simulink library "inp"  (Simulink 7.4)
settings: Solver=ode45  StartTime=0.0  StopTime=10.0  RelTol=1e-3
undefined symbols (not defined in the file): AINP_BrkPedalInterp_X_bar, C_TASK_10MS_S, ENUM_SHIFTER_D, ENUM_SHIFTER_N, ENUM_SHIFTER_P, ENUM_SHIFTER_R, KINP_BonnetCloseVehSpdThre_kph, KINP_EDUCoolantTempFilTm_s, KINP_EDUOilPressureFilTm_s, KINP_EDUOilTempFilTm_s, KINP_EDUSynchDisp_mm, KINP_EDUSynchPosnPWMDC_pct_LowerLimit, KINP_EDUSynchPosnPWMDC_pct_ovrdflg, KINP_EDUSynchPosnPWMDC_pct_ovrdval, KINP_EDUSynchPosnPWMDC_pct_UpperLimit, KINP_ShifterPosConfirmD_s, KINP_ShifterPosConfirmN_s, KINP_ShifterPosConfirmP_s, KINP_ShifterPosConfirmR_s, KINP_SingleAccPedalFltRateLim_pct, KINP_TMSpd2VehSpdSigNeg_rpm, KINP_TMSpd2VehSpdSigPos_rpm, KINP_ValidCheck_EDUSynchPosnPWMDC_dec, KINP_ValidCheck_EDUSynchPosnPWMDC_inc, KINP_ValidCheck_EDUSynchPosnPWMDC_lim, KINP_VehSpdSigKeepThres_kph, KPH2MPS, MIN2SEC, MINP_BrkPedalInterp_pct, MPS2KPH, PI, seat_version_control_block_callbacks, TIRE_RADIUS
libraries: inp_lib x166, hcu_lib x4, simulink x1
(part 1 of 9)
settings Model: Creator=tunfl  LastModifiedBy=tunfl
settings Model: ModifiedHistory=|
  | Function: INP
  | Version: 11.0.9
  | Time: 2012-08-28 16:30:24
  | By: tunfl
  | 0036:ACR_INP_0006:INP: Filter process change about shifter position
  | 
  | 
  | Function: INP
  | Version: 11.0.10
  | Time: 2012-09-03 11:55:18
  | By: tunfl
  | Bug fix for Mantis2038(ACR_INP_0006): Deleted VSRV_ShifterPosValid_ovrdflg&VSRV_ShifterPosValid_ovrdval
  | 
  | 
  | Function: INP
  | Version: 11.0.11
  | Time: 2012-10-10 16:30:31
  | By: tunfl
  | Mantis 2033: Added increasing filter for accelerate pedal position
  | 
  | 
  | Function: INP
  | Version: 11.0.12
  | Time: 2012-10-11 11:20:51
  | By: tunfl
  | Mantis 2079: Newly add signals:VINP_TMOverTemp_flg && VINP_ISGOverTemp_flg
  | 
  | 
  | Function: INP
  | Version: 11.0.13
  | Time: 2012-10-11 11:22:44
  | By: tunfl
  | Mantis 2078: Newly add new signals: VINP_TMDerating_flg && VINP_ISGDerating_flg
  | 
  | 
  | Function: INP
  | Version: 11.0.14
  | Time: 2012-10-16 14:48:04
  | By: tunfl
  | Fixed Library-Link problem for signal: VINP_ShifterPosValid_flg
  | 
  | 
  | Function: INP
  | Version: 11.0.15
  | Time: 2012-10-19 16:16:11
  | By: tunfl
  | Added a new signal: VHAL_ShifterPosProtFault_flg
  | 
  | 
  | Function: INP
  | Version: 11.0.16
  | Time: 2012-11-23 11:36:28
  | By: tunfl
  | Fixed the missing GoTo label problem.
  | 
  | 
  | Function: INP
  | Version: 11.0.17
  | Time: 2012-12-04 09:11:36
  | By: tunfl
  | Changed MAX/MIN value of ISGSpeed to +/-7000
  | 
  | 
  | Function: INP
  | Version: 11.0.18
  | Time: 2013-03-15 10:45:21
  | By: wuqnj
  | Mantis 002142(RSC_INP_0007) and 002147(RSC_INP_0008): New simplification library and CAN MsgActive signals are derived from DSM rather than HAL lay.
  | 
  | 
  | Function: INP
  | Version: 11.0.22
  | Time: 2013-03-19 10:45:50
  | By: wuqnj
  | Add signals into INP fit for v1.7 dbc definition.
  | 
  | 
  | Function: INP
  | Version: 11.0.25
  | Time: 2013-04-10 13:18:30
  | By: wuqnj
  | Add the signals display in INCA for VINP_ISGPwrAct_kW and VINP_ISGOffsetAng_deg
  | 
  | 
  | Function: INP
  | Version: 11.0.26
  | Time: 2013-04-22 16:40:45
  | By: tunfl
  | Changed the improper name of some variables, e.g.  message active signals are started with 'VHAL'
  | 
  | 
  | Function: INP
  | Version: 11.0.28
  | Time: 2013-07-25 13:52:57
  | By: tunfl
  | Mantis_2320: INP/PMM: SCU protection fault should be taken into consideration when determining SCU message is active or not
  | 
  | 
  | Function: INP
  | Version: 11.0.29
  | Time: 2013-08-02 09:13:15
  | By: tunfl
  | Break link with timer library.
  | 
  | 
  | Function: INP
  | Version: 11.0.30
  | Time: 2013-08-05 11:11:04
  | By: tunfl
  | Mantis_2323:INP: Several hardwired signals is processed with first order filter.(EDU Oil pressure, coolant temp, oil temp)

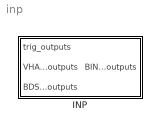
== system inp ==
  INP : Subsystem

== system inp/INP ==
  trig_outputs : Inport
  VHAL_outputs : Inport  Port=2  UseBusObject=on
      settings: BusObject=BHAL_outputs
  BDSM_outputs : Inport  Port=3
  Bus Creator : BusCreator  Inputs=3
  Bus Creator2 : BusCreator  Inputs=5
  Bus Selector : BusSelector  OutputSignals=trig_inp_5ms,trig_inp_10ms,trig_inp_20ms,trig_inp_50ms,trig_inp_100ms
  Bus Selector2 : BusSelector  OutputSignals=VHAL_outputs_5ms,VHAL_outputs_10ms,VHAL_outputs_20ms,VHAL_outputs_50ms,VHAL_outputs_100ms
  Chart : Stateflow chart  RTWFcnName=INP_5MS  RTWFileName=INP
      settings: RTWSystemCode=Function  RTWFcnNameOpts=User specified  RTWFileNameOpts=User specified
  Chart1 : Stateflow chart  RTWFcnName=INP_5MS  RTWFileName=INP
      settings: RTWSystemCode=Inline  RTWFcnNameOpts=User specified  RTWFileNameOpts=User specified
  INP_100MS : Subsystem  TreatAsAtomicUnit=on  RTWFcnName=INP_100MS  RTWFileName=INP
      settings: RTWSystemCode=Function  RTWFcnNameOpts=User specified  RTWFileNameOpts=User specified
  INP_10MS : Subsystem  TreatAsAtomicUnit=on  RTWFcnName=INP_10MS  RTWFileName=INP
      settings: RTWSystemCode=Function  RTWFcnNameOpts=User specified  RTWFileNameOpts=User specified
  INP_20MS : Subsystem  TreatAsAtomicUnit=on  RTWFcnName=INP_20MS  RTWFileName=INP
      settings: RTWSystemCode=Function  RTWFcnNameOpts=User specified  RTWFileNameOpts=User specified
  INP_50MS : Subsystem  TreatAsAtomicUnit=on  RTWFcnName=INP_50MS  RTWFileName=INP
      settings: RTWSystemCode=Function  RTWFcnNameOpts=User specified  RTWFileNameOpts=User specified
  INP_5MS : Subsystem  TreatAsAtomicUnit=on
  INP_MsgAlive_flg : Subsystem  TreatAsAtomicUnit=on  RTWFcnName=INP_MsgAlive_flg  RTWFileName=INP
      settings: RTWSystemCode=Inline  RTWFcnNameOpts=User specified  RTWFileNameOpts=User specified
  Pre-Process : Subsystem
  Version_Control : Subsystem  LoadFcn=seat_version_control_block_callbacks(gcb,'load');  mask(SEAT_Version_Control){version=11.0.30, b_submit_to_excel=on, function_type=Sub, function_name=INP, record_file_name=INP_VersionControl.xlsx, version_on_load=11.0.30, version_last_saved=11.0.30, file_bytes_on_load=1788854, file_date_on_load=735451.46667824069, file_name_on_load=inp.mdl}
      mask prompts: b_submit_to_excel "Submit to record file"; function_type "Function Type"; function_name "Function Name"; record_file_name "Record File"; file_name_on_load "Mask Parameter 11:"
      mask help:
      | Used to record model and software versions for EP11
      | 1. Version display
      | 2. Submit model change to the target record file (file location could be customized in the "Setting" tab)
      settings: ModelCloseFcn=seat_version_control_block_callbacks(gcb,'modelclose')
      mask StyleString: edit,checkbox,popup(Main|Sub),edit,edit,edit,edit,edit,edit,edit
      mask TabNameString: Version,Version,Setting,Setting,Setting,Setting,Setting,Setting,Setting,Setting
      mask Display: disp(sprintf('Function: \t%s\nVersion: \t%s',function_name,version))
  BINP_outputs : Outport  UseBusObject=on
      settings: BusObject=BINP_outputs
  wires:
  [BDSM_outputs] -> Pre-Process/3(BDSM_outputs)
  [trig_can_msg_alive_10ms] -> INP_MsgAlive_flg/Trigger  "fcn_call"
  Chart1/2(trig_can_msg_alive_10ms) -> [trig_can_msg_alive_10ms]
  Chart1/1(trig_inp_raw_10ms) -> [trig_inp_raw_10ms]
  [trig_inp_10ms] -> Chart1/Trigger
  [BINP_CANMsgAlive] -> INP_20MS/2(BINP_CANMsgAlive)
  [BINP_CANMsgAlive] -> INP_50MS/2(BINP_CANMsgAlive)
  [BINP_CANMsgAlive] -> INP_100MS/2(BINP_CANMsgAlive)
  [BINP_CANMsgAlive] -> INP_10MS/2(BINP_CANMsgAlive)
  INP_MsgAlive_flg/1(BINP_CANMsgAlive) -> [BINP_CANMsgAlive]
  BDSM_outputs/1 -> [BDSM_outputs], INP_MsgAlive_flg/1(BDSM_outputs)
  Bus Creator/1 -> [trig_sig_chk]
  Chart/4(trig_sig_chk_100ms) -> Bus Creator/3
  Chart/3(trig_sig_chk_10ms) -> Bus Creator/2
  [trig_sig_chk] -> Pre-Process/1(trig_sig_chk)
  Bus Selector/5 -> [trig_inp_100ms]  "<trig_inp_100ms>"
  Bus Selector/4 -> [trig_inp_50ms]  "<trig_inp_50ms>"
  Bus Selector/3 -> [trig_inp_20ms]  "<trig_inp_20ms>"
  Bus Selector/2 -> [trig_inp_10ms]  "<trig_inp_10ms>"
  Bus Selector/1 -> [trig_inp_5ms]  "<trig_inp_5ms>"
  trig_outputs/1 -> Bus Selector/1
  VHAL_outputs/1 -> Bus Selector2/1
  Bus Creator2/1 -> Pre-Process/2(BINP_rawoutputs)  "BINP_rawoutputs"
  Pre-Process/1(BINP_outputs) -> BINP_outputs/1  "BINP_outputs"
  [trig_inp_100ms] -> INP_100MS/Trigger
  [trig_inp_50ms] -> INP_50MS/Trigger
  [trig_inp_20ms] -> INP_20MS/Trigger
  [trig_inp_raw_10ms] -> INP_10MS/Trigger
  Bus Selector2/1 -> INP_5MS/1(BHAL_IN5MS)  "<VHAL_outputs_5ms>"
  INP_5MS/1(BINP_rawoutputs_5ms) -> Bus Creator2/1
  INP_100MS/1(BINP_rawoutputs_100ms) -> Bus Creator2/5
  INP_50MS/1(BINP_rawoutputs_50ms) -> Bus Creator2/4
  INP_20MS/1(BINP_rawoutputs_20ms) -> Bus Creator2/3
  INP_10MS/1(BINP_rawoutputs_10ms) -> Bus Creator2/2
  Bus Selector2/5 -> INP_100MS/1(BHAL_IN_100ms)  "<VHAL_outputs_100ms>"
  Bus Selector2/4 -> INP_50MS/1(BHAL_IN_50ms)  "<VHAL_outputs_50ms>"
  Bus Selector2/3 -> INP_20MS/1(BHAL_IN_20ms)  "<VHAL_outputs_20ms>"
  Bus Selector2/2 -> INP_10MS/1(BHAL_IN_10ms)  "<VHAL_outputs_10ms>"
  Chart/1(trig_5ms_raw) -> [trig_5ms_raw]
  Chart/2(trig_sig_chk_5ms) -> Bus Creator/1
  [trig_5ms_raw] -> INP_5MS/Trigger
  [trig_inp_5ms] -> Chart/Trigger

== system inp/INP/INP_100MS ==
  BHAL_IN_100ms : Inport  OutDataType=fixdt(1, 16)  OutScaling=2^0
  BINP_CANMsgAlive : Inport  Port=2  OutDataType=fixdt(1, 16)  OutScaling=2^0
  INP_100MS_fcn_call : TriggerPort  TriggerType=function-call
  BSRV_In_ovrdflgs : Subsystem
  BSRV_in_ovrdvals : Subsystem
  Bus Creator3 : BusCreator  Inputs=9
  Bus Selector1 : BusSelector  OutputSignals=VINP_ISCMsgAlive_flg
  Bus Selector14 : BusSelector  OutputSignals=VINP_SMUMsgAlive_flg
  Bus Selector3 : BusSelector  OutputSignals=VINP_TCMsgAlive_flg
  Bus Selector4 : BusSelector  OutputSignals=VINP_ISCMsgAlive_flg
  Bus Selector5 : BusSelector  OutputSignals=VINP_ISCMsgAlive_flg
  Bus Selector7 : BusSelector  OutputSignals=VINP_PMUMsgAlive_flg
  Bus Selector8 : BusSelector  OutputSignals=VINP_SMUMsgAlive_flg
  Bus Selector9 : BusSelector  OutputSignals=VINP_SMUMsgAlive_flg
  HW_HCU_100ms : Subsystem
  Message (100ms) ISC_HSC2_FrP01 : Subsystem
  Message (100ms) ISC_HSC2_FrP02 : Subsystem
  Message (100ms) ISC_HSC2_FrP05 : Subsystem
  Message (100ms) PMU_HSC_FrP00 : Subsystem
  Message (100ms) SMU_HSC_FrP06 : Subsystem
  Message (100ms) SMU_HSC_FrP07 : Subsystem
  Message (100ms) TC_HSC2_FrP03 : Subsystem
  Message (90ms) SMU_HSC_FrP00 : Subsystem
  BINP_rawoutputs_100ms : Outport  OutDataType=fixdt(1, 16)  OutScaling=2^0
  wires:
  [MsgAlive] -> Bus Selector14/1
  [MsgAlive] -> Bus Selector9/1
  [MsgAlive] -> Bus Selector8/1
  [MsgAlive] -> Bus Selector7/1
  [MsgAlive] -> Bus Selector5/1
  [MsgAlive] -> Bus Selector4/1
  [MsgAlive] -> Bus Selector3/1
  [MsgAlive] -> Bus Selector1/1
  BINP_CANMsgAlive/1 -> [MsgAlive]
  Bus Selector5/1 -> Message (100ms) ISC_HSC2_FrP02/4(VINP_ISCMsgAlive_flg)  "<VINP_ISCMsgAlive_flg>"
  HW_HCU_100ms/1(BINP_HW_HCU_100ms) -> Bus Creator3/9
  [BSRV_In_ovrdvals] -> HW_HCU_100ms/3(BSRV_In_ovrdvals)
  [BSRV_In_ovrdflgs] -> HW_HCU_100ms/2(BSRV_In_ovrdflgs)
  Message (90ms) SMU_HSC_FrP00/1(BINP_SMU_HSC_FrP00) -> Bus Creator3/8
  Message (100ms) SMU_HSC_FrP07/1(BINP_SMU_HSC_FrP07) -> Bus Creator3/7
  Message (100ms) SMU_HSC_FrP06/1(BINP_SMU_HSC_FrP06) -> Bus Creator3/6
  Message (100ms) PMU_HSC_FrP00/1(BINP_PMU_HSC_FrP00) -> Bus Creator3/5
  BSRV_in_ovrdvals/1(output_bus) -> [BSRV_In_ovrdvals]
  BSRV_In_ovrdflgs/1(output_bus) -> [BSRV_In_ovrdflgs]
  Bus Creator3/1 -> BINP_rawoutputs_100ms/1  "BINP_rawoutputs_100ms"
  [BSRV_In_ovrdvals] -> Message (100ms) SMU_HSC_FrP07/3(BSRV_In_ovrdvals)
  [BSRV_In_ovrdflgs] -> Message (100ms) SMU_HSC_FrP07/2(BSRV_In_ovrdflgs)
  Bus Selector9/1 -> Message (100ms) SMU_HSC_FrP07/4(VINP_SMUMsgAlive_flg)  "<VINP_SMUMsgAlive_flg>"
  [BSRV_In_ovrdvals] -> Message (100ms) SMU_HSC_FrP06/3(BSRV_In_ovrdvals)
  [BSRV_In_ovrdflgs] -> Message (100ms) SMU_HSC_FrP06/2(BSRV_In_ovrdflgs)
  Bus Selector8/1 -> Message (100ms) SMU_HSC_FrP06/4(VINP_SMUMsgAlive_flg)  "<VINP_SMUMsgAlive_flg>"
  Bus Selector7/1 -> Message (100ms) PMU_HSC_FrP00/4(VINP_PMUMsgAlive_flg)  "<VINP_PMUMsgAlive_flg>"
  [BSRV_In_ovrdvals] -> Message (100ms) PMU_HSC_FrP00/3(BSRV_In_ovrdvals)
  [BSRV_In_ovrdflgs] -> Message (100ms) PMU_HSC_FrP00/2(BSRV_In_ovrdflgs)
  [BSRV_In_ovrdvals] -> Message (100ms) ISC_HSC2_FrP02/3(BSRV_In_ovrdvals)
  [BSRV_In_ovrdflgs] -> Message (100ms) ISC_HSC2_FrP02/2(BSRV_In_ovrdflgs)
  [BSRV_In_ovrdvals] -> Message (100ms) ISC_HSC2_FrP01/3(BSRV_In_ovrdvals)
  [BSRV_In_ovrdflgs] -> Message (100ms) ISC_HSC2_FrP01/2(BSRV_In_ovrdflgs)
  Bus Selector4/1 -> Message (100ms) ISC_HSC2_FrP01/4(VINP_ISCMsgAlive_flg)  "<VINP_ISCMsgAlive_flg>"
  [BSRV_In_ovrdvals] -> Message (100ms) TC_HSC2_FrP03/3(BSRV_In_ovrdvals)
  [BSRV_In_ovrdflgs] -> Message (100ms) TC_HSC2_FrP03/2(BSRV_In_ovrdflgs)
  Bus Selector3/1 -> Message (100ms) TC_HSC2_FrP03/4(VINP_TCMsgAlive_flg)  "<VINP_TCMsgAlive_flg>"
  Bus Selector1/1 -> Message (100ms) ISC_HSC2_FrP05/4(VINP_ISCMsgAlive_flg)  "<VINP_ISCMsgAlive_flg>"
  [BSRV_In_ovrdvals] -> Message (100ms) ISC_HSC2_FrP05/3(BSRV_In_ovrdvals)
  [BSRV_In_ovrdflgs] -> Message (100ms) ISC_HSC2_FrP05/2(BSRV_In_ovrdflgs)
  Bus Selector14/1 -> Message (90ms) SMU_HSC_FrP00/4(VINP_SMUMsgAlive_flg)  "<VINP_SMUMsgAlive_flg>"
  [BSRV_In_ovrdflgs] -> Message (90ms) SMU_HSC_FrP00/2(BSRV_In_ovrdflgs)
  [BSRV_In_ovrdvals] -> Message (90ms) SMU_HSC_FrP00/3(BSRV_In_ovrdvals)
  Message (100ms) ISC_HSC2_FrP05/1(BINP_ISC_HSC2_FrP05) -> Bus Creator3/1
  Message (100ms) TC_HSC2_FrP03/1(BINP_TC_HSC2_FrP03) -> Bus Creator3/2
  Message (100ms) ISC_HSC2_FrP01/1(BINP_ISC_HSC2_FrP01) -> Bus Creator3/3
  Message (100ms) ISC_HSC2_FrP02/1(BINP_ISC_HSC2_FrP02) -> Bus Creator3/4
  BHAL_IN_100ms/1 -> HW_HCU_100ms/1(BHAL_IN_100ms), Message (90ms) SMU_HSC_FrP00/1(BHAL_IN_100ms), Message (100ms) SMU_HSC_FrP07/1(BHAL_IN_100ms), Message (100ms) SMU_HSC_FrP06/1(BHAL_IN_100ms), Message (100ms) PMU_HSC_FrP00/1(BHAL_IN_100ms), Message (100ms) ISC_HSC2_FrP02/1(BHAL_IN_100ms), Message (100ms) ISC_HSC2_FrP01/1(BHAL_IN_100ms), Message (100ms) TC_HSC2_FrP03/1(BHAL_IN_100ms), Message (100ms) ISC_HSC2_FrP05/1(BHAL_IN_100ms)

== system inp/INP/INP_10MS ==
  BHAL_IN_10ms : Inport  OutDataType=fixdt(1, 16)  OutScaling=2^0
  BINP_CANMsgAlive : Inport  Port=2  OutDataType=fixdt(1, 16)  OutScaling=2^0
  INP_10MS_fcn_call : TriggerPort  TriggerType=function-call
  BSRV_in_ovrdflgs : Subsystem
  BSRV_in_ovrdvals : Subsystem
  Bus Creator : BusCreator  Inputs=12
  Bus Selector1 : BusSelector  OutputSignals=VINP_ISCMsgAlive_flg
  Bus Selector{5,8..9,11} (4 alike) : BusSelector  OutputSignals=VINP_DSCMsgAlive_flg
  Bus Selector12 : BusSelector  OutputSignals=VINP_TCMsgAlive_flg
  Bus Selector13 : BusSelector  OutputSignals=VINP_ISCMsgAlive_flg
  Bus Selector2 : BusSelector  OutputSignals=VINP_TCMsgAlive_flg
  Bus Selector3 : BusSelector  OutputSignals=VINP_EMSMsgAlive_flg
  Bus Selector4 : BusSelector  OutputSignals=VINP_EMSMsgAlive_flg
  Bus Selector7 : BusSelector  OutputSignals=VINP_SCUMsgAlive_flg
  HW_HCU_10ms : Subsystem
  Message (10ms) ABS_DSC_HSC_FrP00 : Subsystem
  Message (10ms) ABS_DSC_HSC_FrP03 : Subsystem
  Message (10ms) EMS_HSC_FrP00 : Subsystem
  Message (10ms) EMS_HSC_FrP07 : Subsystem
  Message (10ms) ISC_HSC2_FrP03 : Subsystem
  Message (10ms) ISC_HSC2_FrP04 : Subsystem
  Message (10ms) SCU_HSC_FrP00 : Subsystem
  Message (10ms) TC_HSC2_FrP01 : Subsystem
  Message (10ms) TC_HSC2_FrP02 : Subsystem
  Message (10ms)DSC_HSC_FrP00 : Subsystem
  Message (10ms)DSC_HSC_FrP02 : Subsystem
  BINP_rawoutputs_10ms : Outport  OutDataType=fixdt(1, 16)  OutScaling=2^0
  wires:
  [MsgAlive] -> Bus Selector1/1
  [MsgAlive] -> Bus Selector5/1
  [MsgAlive] -> Bus Selector8/1
  [MsgAlive] -> Bus Selector9/1
  [MsgAlive] -> Bus Selector7/1
  [MsgAlive] -> Bus Selector11/1
  [MsgAlive] -> Bus Selector12/1
  [MsgAlive] -> Bus Selector13/1
  [MsgAlive] -> Bus Selector4/1
  [MsgAlive] -> Bus Selector3/1
  [MsgAlive] -> Bus Selector2/1
  BINP_CANMsgAlive/1 -> [MsgAlive]
  HW_HCU_10ms/1(BINP_HW_HCU_10ms) -> Bus Creator/12
  [BSRV_In_ovrdvals] -> HW_HCU_10ms/3(BSRV_In_ovrdvals)
  [BSRV_In_ovrdflgs] -> HW_HCU_10ms/2(BSRV_In_ovrdflgs)
  Bus Selector3/1 -> Message (10ms) EMS_HSC_FrP00/4(VINP_EMSMsgAlive_flg)  "<VINP_EMSMsgAlive_flg>"
  [BSRV_In_ovrdvals] -> Message (10ms) EMS_HSC_FrP00/3(BSRV_In_ovrdvals)
  [BSRV_In_ovrdflgs] -> Message (10ms) EMS_HSC_FrP00/2(BSRV_In_ovrdflgs)
  Message (10ms) ISC_HSC2_FrP04/1(BINP_ISC_HSC2_FrP04) -> Bus Creator/11
  Message (10ms) ISC_HSC2_FrP03/1(BINP_ISC_HSC2_FrP03) -> Bus Creator/10
  Message (10ms) TC_HSC2_FrP01/1(BINP_TC_HSC2_FrP01) -> Bus Creator/9
  Message (10ms) ABS_DSC_HSC_FrP03/1(BINP_ABS_DSC_HSC_FrP03) -> Bus Creator/8
  Message (10ms) SCU_HSC_FrP00/1(BINP_SCU_HSC_FrP00) -> Bus Creator/7
  Message (10ms)DSC_HSC_FrP02/1(BINP_DSC_HSC_FrP02) -> Bus Creator/6
  Message (10ms)DSC_HSC_FrP00/1(BINP_DSC_HSC_FrP00) -> Bus Creator/5
  Message (10ms) ABS_DSC_HSC_FrP00/1(BINP_ABS_DSC_HSC_FrP00) -> Bus Creator/4
  Message (10ms) EMS_HSC_FrP07/1(BINP_EMS_HSC_FrP07) -> Bus Creator/3  "BINP_EMS_HSC_FrP07"
  Message (10ms) EMS_HSC_FrP00/1(BINP_EMS_HSC_FrP00) -> Bus Creator/2
  Message (10ms) TC_HSC2_FrP02/1(BINP_TC_HSC2_FrP02) -> Bus Creator/1
  Bus Selector5/1 -> Message (10ms) ABS_DSC_HSC_FrP00/4(VINP_DSCMsgAlive_flg)  "<VINP_DSCMsgAlive_flg>"
  [BSRV_In_ovrdflgs] -> Message (10ms) ABS_DSC_HSC_FrP00/2(BSRV_In_ovrdflgs)
  [BSRV_In_ovrdvals] -> Message (10ms) ABS_DSC_HSC_FrP00/3(BSRV_In_ovrdvals)
  Bus Selector8/1 -> Message (10ms)DSC_HSC_FrP00/4(VINP_DSCMsgAlive_flg)  "<VINP_DSCMsgAlive_flg>"
  [BSRV_In_ovrdflgs] -> Message (10ms)DSC_HSC_FrP00/2(BSRV_In_ovrdflgs)
  [BSRV_In_ovrdvals] -> Message (10ms)DSC_HSC_FrP00/3(BSRV_In_ovrdvals)
  BSRV_in_ovrdvals/1(output_bus) -> [BSRV_In_ovrdvals]
  BSRV_in_ovrdflgs/1(output_bus) -> [BSRV_In_ovrdflgs]
  Bus Selector13/1 -> Message (10ms) ISC_HSC2_FrP03/4(VINP_ISCMsgAlive_flg)  "<VINP_ISCMsgAlive_flg>"
  [BSRV_In_ovrdflgs] -> Message (10ms) ISC_HSC2_FrP03/2(BSRV_In_ovrdflgs)
  [BSRV_In_ovrdvals] -> Message (10ms) ISC_HSC2_FrP03/3(BSRV_In_ovrdvals)
  Bus Selector12/1 -> Message (10ms) TC_HSC2_FrP01/4(VINP_TCMsgAlive_flg)  "<VINP_TCMsgAlive_flg>"
  [BSRV_In_ovrdflgs] -> Message (10ms) TC_HSC2_FrP01/2(BSRV_In_ovrdflgs)
  [BSRV_In_ovrdvals] -> Message (10ms) TC_HSC2_FrP01/3(BSRV_In_ovrdvals)
  Bus Selector11/1 -> Message (10ms) ABS_DSC_HSC_FrP03/4(VINP_DSCMsgAlive_flg)  "<VINP_DSCMsgAlive_flg>"
  [BSRV_In_ovrdflgs] -> Message (10ms) ABS_DSC_HSC_FrP03/2(BSRV_In_ovrdflgs)
  [BSRV_In_ovrdvals] -> Message (10ms) ABS_DSC_HSC_FrP03/3(BSRV_In_ovrdvals)
  BHAL_IN_10ms/1 -> HW_HCU_10ms/1(BHAL_IN_10ms), Message (10ms) ISC_HSC2_FrP04/1(BHAL_IN_10ms), Message (10ms) ISC_HSC2_FrP03/1(BHAL_IN_10ms), Message (10ms) TC_HSC2_FrP01/1(BHAL_IN_10ms), Message (10ms) ABS_DSC_HSC_FrP03/1(BHAL_IN_10ms), Message (10ms) SCU_HSC_FrP00/1(BHAL_IN_10ms), Message (10ms)DSC_HSC_FrP02/1(BHAL_IN_10ms), Message (10ms)DSC_HSC_FrP00/1(BHAL_IN_10ms), Message (10ms) ABS_DSC_HSC_FrP00/1(BHAL_IN_10ms), Message (10ms) EMS_HSC_FrP07/1(BHAL_IN_10ms), Message (10ms) EMS_HSC_FrP00/1(BHAL_IN_10ms), Message (10ms) TC_HSC2_FrP02/1(BHAL_IN_10ms)
  Bus Creator/1 -> BINP_rawoutputs_10ms/1  "BINP_rawoutputs_10ms"
  Bus Selector2/1 -> Message (10ms) TC_HSC2_FrP02/4(VINP_TCMsgAlive_flg)  "<VINP_TCMsgAlive_flg>"
  [BSRV_In_ovrdflgs] -> Message (10ms) TC_HSC2_FrP02/2(BSRV_In_ovrdflgs)
  [BSRV_In_ovrdvals] -> Message (10ms) TC_HSC2_FrP02/3(BSRV_In_ovrdvals)
  Bus Selector7/1 -> Message (10ms) SCU_HSC_FrP00/4(VINP_SCUMsgAlive_flg)  "<VINP_SCUMsgAlive_flg>"
  [BSRV_In_ovrdflgs] -> Message (10ms) SCU_HSC_FrP00/2(BSRV_In_ovrdflgs)
  [BSRV_In_ovrdvals] -> Message (10ms) SCU_HSC_FrP00/3(BSRV_In_ovrdvals)
  Bus Selector9/1 -> Message (10ms)DSC_HSC_FrP02/4(VINP_DSCMsgAlive_flg)  "<VINP_DSCMsgAlive_flg>"
  [BSRV_In_ovrdflgs] -> Message (10ms)DSC_HSC_FrP02/2(BSRV_In_ovrdflgs)
  [BSRV_In_ovrdvals] -> Message (10ms)DSC_HSC_FrP02/3(BSRV_In_ovrdvals)
  Bus Selector1/1 -> Message (10ms) ISC_HSC2_FrP04/4(VINP_ISCMsgAlive_flg)  "<VINP_ISCMsgAlive_flg>"
  [BSRV_In_ovrdflgs] -> Message (10ms) ISC_HSC2_FrP04/2(BSRV_In_ovrdflgs)
  [BSRV_In_ovrdvals] -> Message (10ms) ISC_HSC2_FrP04/3(BSRV_In_ovrdvals)
  [BSRV_In_ovrdflgs] -> Message (10ms) EMS_HSC_FrP07/2(BSRV_In_ovrdflgs)
  [BSRV_In_ovrdvals] -> Message (10ms) EMS_HSC_FrP07/3(BSRV_In_ovrdvals)
  Bus Selector4/1 -> Message (10ms) EMS_HSC_FrP07/4(VINP_EMSMsgAlive_flg)  "<VINP_EMSMsgAlive_flg>"

== system inp/INP/INP_20MS ==
  BHAL_IN_20ms : Inport  OutDataType=fixdt(1, 16)  OutScaling=2^0
  BINP_CANMsgAlive : Inport  Port=2  OutDataType=fixdt(1, 16)  OutScaling=2^0
  INP_20MS_fcn_call : TriggerPort  TriggerType=function-call
  BSRV_In_ovrdflgs : Subsystem
  BSRV_in_ovrdvals : Subsystem
  Bus Creator : BusCreator  Inputs=8
  Bus Selector1 : BusSelector  OutputSignals=VINP_SMUMsgAlive_flg
  Bus Selector2 : BusSelector  OutputSignals=VINP_EPBMsgAlive_flg
  Bus Selector3 : BusSelector  OutputSignals=VINP_EMSMsgAlive_flg
  Bus Selector4 : BusSelector  OutputSignals=VINP_DSCMsgAlive_flg
  Bus Selector5 : BusSelector  OutputSignals=VINP_BMSMsgAlive_flg
  Bus Selector6 : BusSelector  OutputSignals=VINP_EMSMsgAlive_flg
  Bus Selector8 : BusSelector  OutputSignals=VINP_BMSMsgAlive_flg
  HW_HCU_20ms : Subsystem
  Message (15ms) EMS_HSC_FrP03 : Subsystem
  Message (20ms) BMS_HSC2_FrP03 : Subsystem
  Message (20ms) BMS_HSC2_FrP09 : Subsystem
  Message (20ms) DSC_HSC_FrP04 : Subsystem
  Message (20ms) EMS_HSC_FrP01 : Subsystem
  Message (20ms) EPB_HSC_FrP00 : Subsystem
  Message (20ms) SMU_HSC_FrP02 : Subsystem
  BINP_rawoutputs_20ms : Outport  OutDataType=fixdt(1, 16)  OutScaling=2^0
  wires:
  Message (20ms) BMS_HSC2_FrP09/1(BINP_BMS_HSC2_FrP09) -> Bus Creator/7
  [MsgAlive] -> Bus Selector5/1
  Bus Selector5/1 -> Message (20ms) BMS_HSC2_FrP09/4(VINP_BMSMsgAlive_flg)  "<VINP_BMSMsgAlive_flg>"
  [BSRV_In_ovrdvals] -> Message (20ms) BMS_HSC2_FrP09/3(BSRV_In_ovrdvals)
  [BSRV_In_ovrdflgs] -> Message (20ms) BMS_HSC2_FrP09/2(BSRV_In_ovrdflgs)
  [MsgAlive] -> Bus Selector8/1
  [MsgAlive] -> Bus Selector6/1
  [MsgAlive] -> Bus Selector4/1
  [MsgAlive] -> Bus Selector3/1
  [MsgAlive] -> Bus Selector2/1
  [MsgAlive] -> Bus Selector1/1
  BINP_CANMsgAlive/1 -> [MsgAlive]
  BSRV_In_ovrdflgs/1(output_bus) -> [BSRV_In_ovrdflgs]
  BSRV_in_ovrdvals/1(output_bus) -> [BSRV_In_ovrdvals]
  [BSRV_In_ovrdvals] -> Message (20ms) BMS_HSC2_FrP03/3(BSRV_In_ovrdvals)
  [BSRV_In_ovrdflgs] -> Message (20ms) BMS_HSC2_FrP03/2(BSRV_In_ovrdflgs)
  Bus Selector8/1 -> Message (20ms) BMS_HSC2_FrP03/4(VINP_BMSMsgAlive_flg)  "<VINP_BMSMsgAlive_flg>"
  Bus Selector4/1 -> Message (20ms) DSC_HSC_FrP04/4(VINP_DSCMsgAlive_flg)  "<VINP_DSCMsgAlive_flg>"
  [BSRV_In_ovrdflgs] -> Message (20ms) DSC_HSC_FrP04/2(BSRV_In_ovrdflgs)
  [BSRV_In_ovrdvals] -> Message (20ms) DSC_HSC_FrP04/3(BSRV_In_ovrdvals)
  Bus Selector3/1 -> Message (20ms) EMS_HSC_FrP01/4(VINP_EMSMsgAlive_flg)  "<VINP_EMSMsgAlive_flg>"
  [BSRV_In_ovrdflgs] -> Message (20ms) EMS_HSC_FrP01/2(BSRV_In_ovrdflgs)
  [BSRV_In_ovrdvals] -> Message (20ms) EMS_HSC_FrP01/3(BSRV_In_ovrdvals)
  Bus Selector2/1 -> Message (20ms) EPB_HSC_FrP00/4(VINP_EPBMsgAlive_flg)  "<VINP_EPBMsgAlive_flg>"
  [BSRV_In_ovrdflgs] -> Message (20ms) EPB_HSC_FrP00/2(BSRV_In_ovrdflgs)
  [BSRV_In_ovrdvals] -> Message (20ms) EPB_HSC_FrP00/3(BSRV_In_ovrdvals)
  Bus Selector1/1 -> Message (20ms) SMU_HSC_FrP02/4(VINP_SMUMsgAlive_flg)  "<VINP_SMUMsgAlive_flg>"
  [BSRV_In_ovrdflgs] -> Message (20ms) SMU_HSC_FrP02/2(BSRV_In_ovrdflgs)
  [BSRV_In_ovrdvals] -> Message (20ms) SMU_HSC_FrP02/3(BSRV_In_ovrdvals)
  BHAL_IN_20ms/1 -> Message (20ms) BMS_HSC2_FrP03/1(BHAL_IN_20ms), Message (20ms) BMS_HSC2_FrP09/1(BHAL_IN_20ms), HW_HCU_20ms/1(BHAL_IN_20ms), Message (15ms) EMS_HSC_FrP03/1(BHAL_IN_20ms), Message (20ms) DSC_HSC_FrP04/1(BHAL_IN_20ms), Message (20ms) EMS_HSC_FrP01/1(BHAL_IN_20ms), Message (20ms) EPB_HSC_FrP00/1(BHAL_IN_20ms), Message (20ms) SMU_HSC_FrP02/1(BHAL_IN_20ms)
  Bus Creator/1 -> BINP_rawoutputs_20ms/1  "BINP_rawoutputs_20ms"
  [BSRV_In_ovrdvals] -> Message (15ms) EMS_HSC_FrP03/3(BSRV_In_ovrdvals)
  [BSRV_In_ovrdflgs] -> Message (15ms) EMS_HSC_FrP03/2(BSRV_In_ovrdflgs)
  Bus Selector6/1 -> Message (15ms) EMS_HSC_FrP03/4(VINP_EMSMsgAlive_flg)  "<VINP_EMSMsgAlive_flg>"
  Message (20ms) SMU_HSC_FrP02/1(BINP_SMU_HSC_FrP02) -> Bus Creator/1
  Message (20ms) EPB_HSC_FrP00/1(BINP_EPB_HSC_FrP00) -> Bus Creator/2
  Message (20ms) EMS_HSC_FrP01/1(BINP_EMS_HSC_FrP01) -> Bus Creator/3
  Message (20ms) DSC_HSC_FrP04/1(BINP_DSC_HSC_FrP04) -> Bus Creator/4
  Message (15ms) EMS_HSC_FrP03/1(BINP_EMS_HSC_FrP03) -> Bus Creator/5
  Message (20ms) BMS_HSC2_FrP03/1(BINP_BMS_HSC2_FrP03) -> Bus Creator/6
  [BSRV_In_ovrdflgs] -> HW_HCU_20ms/2(BSRV_In_ovrdflgs)
  [BSRV_In_ovrdvals] -> HW_HCU_20ms/3(BSRV_In_ovrdvals)
  HW_HCU_20ms/1(BINP_HW_HCU_20ms) -> Bus Creator/8

== system inp/INP/INP_50MS ==
  BHAL_IN_50ms : Inport  OutDataType=fixdt(1, 16)  OutScaling=2^0
  BINP_CANMsgAlive : Inport  Port=2  OutDataType=fixdt(1, 16)  OutScaling=2^0
  INP_50MS_fcn_call : TriggerPort  TriggerType=function-call
  BSRV_In_ovrdflgs : Subsystem
  BSRV_in_ovrdvals : Subsystem
  Bus Creator : BusCreator
  Bus Selector1 : BusSelector  OutputSignals=VINP_BMSMsgAlive_flg
  Bus Selector2 : BusSelector  OutputSignals=VINP_SMUMsgAlive_flg
  Bus Selector3 : BusSelector  OutputSignals=VINP_BMSMsgAlive_flg
  Bus Selector7 : BusSelector  OutputSignals=VINP_BMSMsgAlive_flg
  Message (50ms) BMS_HSC2_FrP01 : Subsystem
  Message (50ms) BMS_HSC2_FrP02 : Subsystem
  Message (50ms) BMS_HSC2_FrP05 : Subsystem
  Message (50ms) SMU_HSC_FrP03 : Subsystem
  BINP_rawoutputs_50ms : Outport  OutDataType=fixdt(1, 16)  OutScaling=2^0
  wires:
  [MsgAlive] -> Bus Selector3/1
  Bus Selector3/1 -> Message (50ms) BMS_HSC2_FrP05/4(VINP_BMSMsgAlive_flg)  "<VINP_BMSMsgAlive_flg>"
  [BSRV_In_ovrdflgs] -> Message (50ms) BMS_HSC2_FrP05/2(BSRV_In_ovrdflgs)
  [BSRV_In_ovrdvals] -> Message (50ms) BMS_HSC2_FrP05/3(BSRV_In_ovrdvals)
  Message (50ms) BMS_HSC2_FrP05/1(BINP_BMS_HSC_FrP05) -> Bus Creator/4
  [MsgAlive] -> Bus Selector1/1
  [MsgAlive] -> Bus Selector7/1
  [MsgAlive] -> Bus Selector2/1
  BINP_CANMsgAlive/1 -> [MsgAlive]
  BSRV_In_ovrdflgs/1(output_bus) -> [BSRV_In_ovrdflgs]
  BSRV_in_ovrdvals/1(output_bus) -> [BSRV_In_ovrdvals]
  [BSRV_In_ovrdflgs] -> Message (50ms) BMS_HSC2_FrP01/2(BSRV_In_ovrdflgs)
  [BSRV_In_ovrdvals] -> Message (50ms) BMS_HSC2_FrP01/3(BSRV_In_ovrdvals)
  Bus Creator/1 -> BINP_rawoutputs_50ms/1  "BINP_rawoutputs_50ms"
  [BSRV_In_ovrdflgs] -> Message (50ms) SMU_HSC_FrP03/2(BSRV_In_ovrdflgs)
  [BSRV_In_ovrdvals] -> Message (50ms) SMU_HSC_FrP03/3(BSRV_In_ovrdvals)
  Bus Selector2/1 -> Message (50ms) SMU_HSC_FrP03/4(VINP_SMUMsgAlive_flg)  "<VINP_SMUMsgAlive_flg>"
  BHAL_IN_50ms/1 -> Message (50ms) BMS_HSC2_FrP05/1(BHAL_IN_50ms), Message (50ms) BMS_HSC2_FrP02/1(BHAL_IN_50ms), Message (50ms) BMS_HSC2_FrP01/1(BHAL_IN_50ms), Message (50ms) SMU_HSC_FrP03/1(BHAL_IN_50ms)
  Bus Selector7/1 -> Message (50ms) BMS_HSC2_FrP02/4(VINP_BMSMsgAlive_flg)  "<VINP_BMSMsgAlive_flg>"
  [BSRV_In_ovrdflgs] -> Message (50ms) BMS_HSC2_FrP02/2(BSRV_In_ovrdflgs)
  [BSRV_In_ovrdvals] -> Message (50ms) BMS_HSC2_FrP02/3(BSRV_In_ovrdvals)
  Bus Selector1/1 -> Message (50ms) BMS_HSC2_FrP01/4(VINP_BMSMsgAlive_flg)  "<VINP_BMSMsgAlive_flg>"
  Message (50ms) SMU_HSC_FrP03/1(BINP_SMU_HSC_FrP03) -> Bus Creator/1
  Message (50ms) BMS_HSC2_FrP01/1(BINP_BMS_FrP01) -> Bus Creator/2
  Message (50ms) BMS_HSC2_FrP02/1(BINP_BMS_HSC_FrP02) -> Bus Creator/3

== system inp/INP/INP_5MS ==
  BHAL_IN5MS : Inport  OutDataType=fixdt(1, 16)  OutScaling=2^0
  INP_5MS_fcn_call : TriggerPort  TriggerType=function-call
  BSRV_In_ovrdflgs : Subsystem
  BSRV_in_ovrdvals : Subsystem
  Bus Creator : BusCreator  Inputs=1
  HW_HCU_5ms : Subsystem
  BINP_rawoutputs_5ms : Outport  OutDataType=fixdt(1, 16)  OutScaling=2^0
  wires:
  BSRV_In_ovrdflgs/1(output_bus) -> [BSRV_In_ovrdflgs]
  BSRV_in_ovrdvals/1(output_bus) -> [BSRV_In_ovrdvals]
  BHAL_IN5MS/1 -> HW_HCU_5ms/1(BHAL_outputs)
  [BSRV_In_ovrdflgs] -> HW_HCU_5ms/2(BSRV_In_ovrdflgs)
  [BSRV_In_ovrdvals] -> HW_HCU_5ms/3(BSRV_In_ovrdvals)
  Bus Creator/1 -> BINP_rawoutputs_5ms/1  "BINP_rawoutputs_5ms"
  HW_HCU_5ms/1(BINP_HardwireInputs) -> Bus Creator/1

== system inp/INP/INP_MsgAlive_flg ==
  BDSM_outputs : Inport  OutDataType=fixdt(1, 16)  OutScaling=2^0
  INP_MsgAliveflg_fcn_call : TriggerPort  TriggerType=function-call
  Bus Creator : BusCreator  Inputs=9
  Bus Selector1 : BusSelector  OutputSignals=VDSM_CAN1BusOff_flg,VDSM_CAN2BusOff_flg
  Bus Selector2 : BusSelector  OutputSignals=VDSM_DSCMsgProtnFlt_flg,VDSM_EMSMsgProtnFlt_flg,VDSM_EPBMsgProtnFlt_flg,VDSM_BMSMsgProtnFlt_flg,VDSM_ISCMsgProtnFlt_flg,VDSM_TCMsgProtnFlt_flg,VDSM_SCUMsgProtnFlt_flg
  Bus Selector4 : BusSelector  OutputSignals=VDSM_LosComunictnWthDSC_flg,VDSM_LosComunictnWthEPB_flg,VDSM_LosComunictnWthBMS_flg,VDSM_LosComunictnWthEMS_flg,VDSM_LosComunictnWthISC_flg,VDSM_LosComunictnWthPMU_flg,VDSM_LosComunictnWthSCU_flg,VDSM_LosComunictnWthSMU_flg,VDSM_LosComunictnWthTC_flg
  Logical Operator{1..6,9} (7 alike) : Logic  Operator=NOR  Inputs=3  AllPortsSameDT=off  OutDataTypeMode=boolean  OutDataTypeStr=boolean
  Logical Operator7 : Logic  Operator=NOR  AllPortsSameDT=off  OutDataTypeMode=boolean  OutDataTypeStr=boolean
  Logical Operator8 : Logic  Operator=NOR  AllPortsSameDT=off  OutDataTypeMode=boolean  OutDataTypeStr=boolean
  BINP_CANMsgAlive : Outport  OutDataType=fixdt(1, 16)  OutScaling=2^0
  wires:
  [VDSM_SCUMsgProtnFlt_flg] -> Logical Operator4/3
  Bus Selector2/7 -> [VDSM_SCUMsgProtnFlt_flg]  "<VDSM_SCUMsgProtnFlt_flg>"
  Bus Creator/1 -> BINP_CANMsgAlive/1
  Logical Operator9/1 -> Bus Creator/9  "VINP_TCMsgAlive_flg"
  Logical Operator8/1 -> Bus Creator/8  "VINP_SMUMsgAlive_flg"
  Logical Operator4/1 -> Bus Creator/7  "VINP_SCUMsgAlive_flg"
  Logical Operator7/1 -> Bus Creator/6  "VINP_PMUMsgAlive_flg"
  Logical Operator6/1 -> Bus Creator/5  "VINP_ISCMsgAlive_flg"
  Logical Operator5/1 -> Bus Creator/4  "VINP_EMSMsgAlive_flg"
  Logical Operator3/1 -> Bus Creator/3  "VINP_BMSMsgAlive_flg"
  Logical Operator1/1 -> Bus Creator/2  "VINP_EPBMsgAlive_flg"
  Logical Operator2/1 -> Bus Creator/1  "VINP_DSCMsgAlive_flg"
  [VDSM_CAN1BusOff_flg] -> Logical Operator8/2
  [VDSM_CAN2BusOff_flg] -> Logical Operator9/2
  [VDSM_TCMsgProtnFlt_flg] -> Logical Operator9/3
  Bus Selector4/9 -> Logical Operator9/1  "<VDSM_LosComunictnWthTC_flg>"
  Bus Selector4/8 -> Logical Operator8/1  "<VDSM_LosComunictnWthSMU_flg>"
  [VDSM_CAN1BusOff_flg] -> Logical Operator4/2
  Bus Selector4/7 -> Logical Operator4/1  "<VDSM_LosComunictnWthSCU_flg>"
  Bus Selector4/6 -> Logical Operator7/1  "<VDSM_LosComunictnWthPMU_flg>"
  [VDSM_CAN1BusOff_flg] -> Logical Operator7/2
  Bus Selector4/5 -> Logical Operator6/1  "<VDSM_LosComunictnWthISC_flg>"
  [VDSM_CAN2BusOff_flg] -> Logical Operator6/2
  [VDSM_ISCMsgProtnFlt_flg] -> Logical Operator6/3
  [VDSM_EMSMsgProtnFlt_flg] -> Logical Operator5/3
  Bus Selector4/4 -> Logical Operator5/1  "<VDSM_LosComunictnWthEMS_flg>"
  [VDSM_CAN1BusOff_flg] -> Logical Operator5/2
  [VDSM_CAN2BusOff_flg] -> Logical Operator3/2
  [VDSM_BMSMsgProtnFlt_flg] -> Logical Operator3/3
  Bus Selector4/3 -> Logical Operator3/1  "<VDSM_LosComunictnWthBMS_flg>"
  Bus Selector4/2 -> Logical Operator1/1  "<VDSM_LosComunictnWthEPB_flg>"
  [VDSM_CAN1BusOff_flg] -> Logical Operator1/2
  [VDSM_EPBMsgProtnFlt_flg] -> Logical Operator1/3
  [VDSM_CAN1BusOff_flg] -> Logical Operator2/2
  [VDSM_DSCMsgProtnFlt_flg] -> Logical Operator2/3
  Bus Selector4/1 -> Logical Operator2/1  "<VDSM_LosComunictnWthDSC_flg>"
  Bus Selector2/6 -> [VDSM_TCMsgProtnFlt_flg]  "<VDSM_TCMsgProtnFlt_flg>"
  Bus Selector2/5 -> [VDSM_ISCMsgProtnFlt_flg]  "<VDSM_ISCMsgProtnFlt_flg>"
  Bus Selector2/4 -> [VDSM_BMSMsgProtnFlt_flg]  "<VDSM_BMSMsgProtnFlt_flg>"
  Bus Selector2/3 -> [VDSM_EPBMsgProtnFlt_flg]  "<VDSM_EPBMsgProtnFlt_flg>"
  Bus Selector2/2 -> [VDSM_EMSMsgProtnFlt_flg]  "<VDSM_EMSMsgProtnFlt_flg>"
  Bus Selector2/1 -> [VDSM_DSCMsgProtnFlt_flg]  "<VDSM_DSCMsgProtnFlt_flg>"
  Bus Selector1/2 -> [VDSM_CAN2BusOff_flg]  "<VDSM_CAN2BusOff_flg>"
  Bus Selector1/1 -> [VDSM_CAN1BusOff_flg]  "<VDSM_CAN1BusOff_flg>"
  BDSM_outputs/1 -> Bus Selector2/1, Bus Selector1/1, Bus Selector4/1

== system inp/INP/Pre-Process ==
  trig_sig_chk : Inport  OutDataType=fixdt(1, 16)  OutScaling=2^0
  BINP_rawoutputs : Inport  Port=2  OutDataType=fixdt(1, 16)  OutScaling=2^0
  BDSM_outputs : Inport  Port=3  OutDataType=fixdt(1, 16)  OutScaling=2^0
  BINP_ouputs_100ms : Subsystem
      settings: RTWSystemCode=Inline
  BINP_ouputs_10ms : Subsystem
      settings: RTWSystemCode=Inline
  BINP_ouputs_5ms : Subsystem
      settings: RTWSystemCode=Inline
  Bus Creator : BusCreator  Inputs=5
  Bus Selector : BusSelector  OutputSignals=trig_sig_chk_5ms,trig_sig_chk_10ms,trig_sig_chk_100ms
  Bus Selector1 : BusSelector  OutputSignals=BINP_rawoutputs_10ms
  Bus Selector2 : BusSelector  OutputSignals=BINP_rawoutputs_10ms  OutputAsBus=on
  Bus Selector3 : BusSelector  OutputSignals=BINP_rawoutputs_20ms  OutputAsBus=on
  Bus Selector4 : BusSelector  OutputSignals=BINP_rawoutputs_50ms  OutputAsBus=on
  Bus Selector5 : BusSelector  OutputSignals=BINP_rawoutputs_100ms  OutputAsBus=on
  Bus Selector6 : BusSelector  OutputSignals=BINP_rawoutputs_5ms
  Bus Selector7 : BusSelector  OutputSignals=BINP_outputs_5ms.VINP_EDUOutputShaftSpd_rpm,BINP_outputs_5ms.VINP_EDUOutputShaftSpdValid_flg,BINP_outputs_5ms.VINP_EDUSynchPosnPWMKDC_pct,BINP_outputs_5ms.VINP_EDUSynchPosnPWMKDCValid_flg,BINP_outputs_5ms.VINP_EDUSynchPosn_mm,BINP_outputs_5ms.VINP_EDUSynchPosnValid_flg,BINP_outputs_5ms.VINP_EDUSynchPosnPWMDC_pct,BINP_outputs_5ms.VINP_EDUSynchPosnPWMDCValid_flg,BINP_outputs_10ms.BINP_TC_HSC2_FrP02.VINP_TMTqAvailMin_Nm,BINP_outputs_10ms.BINP_TC_HSC2_FrP02.VINP_TMTqAvailMax_Nm,BINP_outputs_10ms.BINP_TC_HSC2_FrP02.VINP_TMInvtCurr_A,BINP_outputs_10ms.BINP_TC_HSC2_FrP02.VINP_TCHSC2FrP02Active_flg,BINP_outputs_10ms.BINP_EMS_HSC_FrP00.VINP_BrkLightSwitchActive_flg,BINP_outputs_10ms.BINP_EMS_HSC_FrP00.VINP_BrkLightSwitchActiveValid_flg,BINP_outputs_10ms.BINP_EMS_HSC_FrP00.VINP_EngSpd_rpm,BINP_outputs_10ms.BINP_EMS_HSC_FrP00.VINP_EngSpdValid_flg,BINP_outputs_10ms.BINP_EMS_HSC_FrP00.VINP_EngTqFriction_Nm,BINP_outputs_10ms.BINP_EMS_HSC_FrP00.VINP_EngTqIndAct_Nm,BINP_outputs_10ms.BINP_EMS_HSC_FrP00.VINP_EngTqIndActValid_flg,BINP_outputs_10ms.BINP_EMS_HSC_FrP00.VINP_EngTqStandard_Nm,BINP_outputs_10ms.BINP_EMS_HSC_FrP00.VINP_CruiseTqReq_Nm,BINP_outputs_10ms.BINP_EMS_HSC_FrP00.VINP_EngTqModelStatus_enum,BINP_outputs_10ms.BINP_EMS_HSC_FrP00.VINP_KeySwitchStateIGN_flg,BINP_outputs_10ms.BINP_EMS_HSC_FrP00.VINP_EMSHSCFrP00Active_flg,BINP_outputs_10ms.BINP_EMS_HSC_FrP07.VINP_EngSpdMon_rpm,BINP_outputs_10ms.BINP_EMS_HSC_FrP07.VINP_EngStartComplete_flg,BINP_outputs_10ms.BINP_EMS_HSC_FrP07.VINP_EngStopped_flg,BINP_outputs_10ms.BINP_EMS_HSC_FrP07.VINP_EngTqAllowedMinMon_Nm,BINP_outputs_10ms.BINP_EMS_HSC_FrP07.VINP_EngTqMax_Nm,BINP_outputs_10ms.BINP_EMS_HSC_FrP07.VINP_EngTqMin_Nm,BINP_outputs_10ms.BINP_EMS_HSC_FrP07.VINP_FuelCutActive_flg,BINP_outputs_10ms.BINP_EMS_HSC_FrP07.VINP_LamdLoopActive_flg,BINP_outputs_10ms.BINP_EMS_HSC_FrP07.VINP_EngIdle_flg,BINP_outputs_10ms.BINP_EMS_HSC_FrP07.VINP_AccelPedalPosn_pct,BINP_outputs_10ms.BINP_EMS_HSC_FrP07.VINP_AccelPedalPosnValid_flg,BINP_outputs_10ms.BINP_EMS_HSC_FrP07.VINP_EMSFltLevel_enum,BINP_outputs_10ms.BINP_EMS_HSC_FrP07.VINP_CatLightOffReq_flg,BINP_outputs_10ms.BINP_EMS_HSC_FrP07.VINP_EMSHSCFrP07Active_flg,BINP_outputs_10ms.BINP_ABS_DSC_HSC_FrP00.VINP_WheelRoughRoad_mps2,BINP_outputs_10ms.BINP_ABS_DSC_HSC_FrP00.VINP_WheelRoughRoadValid_flg,BINP_outputs_10ms.BINP_ABS_DSC_HSC_FrP00.VINP_ABSDSCHSCFrP00Active_flg,BINP_outputs_10ms.BINP_ABS_DSC_HSC_FrP00.VINP_VehSpd_kph,BINP_outputs_10ms.BINP_ABS_DSC_HSC_FrP00.VINP_VehSpdValid_flg,BINP_outputs_10ms.BINP_DSC_HSC_FrP00.VINP_GearShiftInhDown_flg,BINP_outputs_10ms.BINP_DSC_HSC_FrP00.VINP_GearShiftInhDownValid_flg,BINP_outputs_10ms.BINP_DSC_HSC_FrP00.VINP_GearShiftInhUp_flg,BINP_outputs_10ms.BINP_DSC_HSC_FrP00.VINP_GearShiftInhUpValid_flg,BINP_outputs_10ms.BINP_DSC_HSC_FrP00.VINP_DSCHSCFrP00Active_flg,BINP_outputs_10ms.BINP_DSC_HSC_FrP02.VINP_ESPTqIncControlActive_flg,BINP_outputs_10ms.BINP_DSC_HSC_FrP02.VINP_ESPTqRedControlActive_flg,BINP_outputs_10ms.BINP_DSC_HSC_FrP02.VINP_ESPTqIncSlowReq_Nm,BINP_outputs_10ms.BINP_DSC_HSC_FrP02.VINP_ESPTqRedFastReq_Nm,BINP_outputs_10ms.BINP_DSC_HSC_FrP02.VINP_ESPTqRedSlowReq_Nm,BINP_outputs_10ms.BINP_DSC_HSC_FrP02.VINP_DSCHSCFrP02Active_flg,BINP_outputs_10ms.BINP_SCU_HSC_FrP00.VINP_ShifterFail_flg,BINP_outputs_10ms.BINP_SCU_HSC_FrP00.VINP_ShifterPos_enum,BINP_outputs_10ms.BINP_SCU_HSC_FrP00.VINP_ShifterInit_flg,BINP_outputs_10ms.BINP_SCU_HSC_FrP00.VINP_ShifterPosValid_flg,BINP_outputs_10ms.BINP_SCU_HSC_FrP00.VINP_SCUHSCFrP00Active_flg,BINP_outputs_10ms.BINP_ABS_DSC_HSC_FrP03.VINP_BrkPedalPosn_pct,BINP_outputs_10ms.BINP_ABS_DSC_HSC_FrP03.VINP_BrkPedalPosnValid_flg,BINP_outputs_10ms.BINP_ABS_DSC_HSC_FrP03.VINP_ABSDSCHSCFrP03Active_flg,BINP_outputs_10ms.BINP_TC_HSC2_FrP01.VINP_TMACShortCircReady_flg,BINP_outputs_10ms.BINP_TC_HSC2_FrP01.VINP_TMDiagReq_flg,BINP_outputs_10ms.BINP_TC_HSC2_FrP01.VINP_TMSpdRaw_rpm,BINP_outputs_10ms.BINP_TC_HSC2_FrP01.VINP_TMMode_enum,BINP_outputs_10ms.BINP_TC_HSC2_FrP01.VINP_TMSpd_rpm,BINP_outputs_10ms.BINP_TC_HSC2_FrP01.VINP_TMSpdValid_flg,BINP_outputs_10ms.BINP_TC_HSC2_FrP01.VINP_TMTqAct_Nm,BINP_outputs_10ms.BINP_TC_HSC2_FrP01.VINP_TMTqActValid_flg,BINP_outputs_10ms.BINP_TC_HSC2_FrP01.VINP_TCHSC2FrP01Active_flg,BINP_outputs_10ms.BINP_ISC_HSC2_FrP03.VINP_ISGACShortCircReady_flg,BINP_outputs_10ms.BINP_ISC_HSC2_FrP03.VINP_ISGDiagReq_flg,BINP_outputs_10ms.BINP_ISC_HSC2_FrP03.VINP_ISGMode_enum,BINP_outputs_10ms.BINP_ISC_HSC2_FrP03.VINP_ISGSpd_rpm,BINP_outputs_10ms.BINP_ISC_HSC2_FrP03.VINP_ISGSpdValid_flg,BINP_outputs_10ms.BINP_ISC_HSC2_FrP03.VINP_ISGTqAct_Nm,BINP_outputs_10ms.BINP_ISC_HSC2_FrP03.VINP_ISGTqActValid_flg,BINP_outputs_10ms.BINP_ISC_HSC2_FrP03.VINP_ISCHSC2FrP03Active_flg,BINP_outputs_10ms.BINP_ISC_HSC2_FrP04.VINP_ISGTqAvailMax_Nm,BINP_outputs_10ms.BINP_ISC_HSC2_FrP04.VINP_ISGTqAvailMin_Nm,BINP_outputs_10ms.BINP_ISC_HSC2_FrP04.VINP_ISGSurgeDampActive_flg,BINP_outputs_10ms.BINP_ISC_HSC2_FrP04.VINP_ISGInvtCurr_A,BINP_outputs_10ms.BINP_ISC_HSC2_FrP04.VINP_ISCHSC2FrP04Active_flg,BINP_outputs_10ms.BINP_HW_HCU_10ms.VINP_CrankActive_flg,BINP_outputs_10ms.BINP_HW_HCU_10ms.VINP_IgnitionOn_flg,BINP_outputs_20ms.BINP_SMU_HSC_FrP02.VINP_SecurityKeyValid_flg,BINP_outputs_20ms.BINP_SMU_HSC_FrP02.VINP_SMUHSCFrP02Active_flg,BINP_outputs_20ms.BINP_EPB_HSC_FrP00.VINP_GSensor_g,BINP_outputs_20ms.BINP_EPB_HSC_FrP00.VINP_EPBStatus_enum,BINP_outputs_20ms.BINP_EPB_HSC_FrP00.VINP_EPBHSCFrP00Active_flg,BINP_outputs_20ms.BINP_EMS_HSC_FrP01.VINP_EngCoolantTemp_C,BINP_outputs_20ms.BINP_EMS_HSC_FrP01.VINP_EngCoolantTempValid_flg,BINP_outputs_20ms.BINP_EMS_HSC_FrP01.VINP_EngIdleTypeReq_enum,BINP_outputs_20ms.BINP_EMS_HSC_FrP01.VINP_CruiseControlActive_flg,BINP_outputs_20ms.BINP_EMS_HSC_FrP01.VINP_EMSHSCFrP01Active_flg,BINP_outputs_20ms.BINP_DSC_HSC_FrP04.VINP_BrkVacPumpState_enum,BINP_outputs_20ms.BINP_DSC_HSC_FrP04.VINP_ESPRegenFault_flg,BINP_outputs_20ms.BINP_DSC_HSC_FrP04.VINP_ESPRegenTargetAtWheel_Nm,BINP_outputs_20ms.BINP_DSC_HSC_FrP04.VINP_DSCHSCFrP04Active_flg,BINP_outputs_20ms.BINP_EMS_HSC_FrP03.VINP_EngAutoStopInhibit_flg,BINP_outputs_20ms.BINP_EMS_HSC_FrP03.VINP_AccPedSingleFlt_flg,BINP_outputs_20ms.BINP_EMS_HSC_FrP03.VINP_AccPedFlt_flg,BINP_outputs_20ms.BINP_EMS_HSC_FrP03.VINP_EngStartReq_enum,BINP_outputs_20ms.BINP_EMS_HSC_FrP03.VINP_EMSHSCFrP03Active_flg,BINP_outputs_20ms.BINP_BMS_HSC2_FrP03.VINP_HVBattChargeCurrMax_A,BINP_outputs_20ms.BINP_BMS_HSC2_FrP03.VINP_HVBattEnergyAvail_kWh,BINP_outputs_20ms.BINP_BMS_HSC2_FrP03.VINP_HVBattBalanceReq_flg,BINP_outputs_20ms.BINP_BMS_HSC2_FrP03.VINP_HVBattFltLampOnReq_flg,BINP_outputs_20ms.BINP_BMS_HSC2_FrP03.VINP_HVBattDisChargeCurrMax_A,BINP_outputs_20ms.BINP_BMS_HSC2_FrP03.VINP_BMSHSC2FrP03Active_flg,BINP_outputs_50ms.BINP_SMU_HSC_FrP03.VINP_AmbientTemp_C,BINP_outputs_50ms.BINP_SMU_HSC_FrP03.VINP_KeySwitchStateCRK_flg,BINP_outputs_50ms.BINP_SMU_HSC_FrP03.VINP_SMUHSCFrP03Active_flg,BINP_outputs_50ms.BINP_BMS_FrP01.VINP_HVBattIsolationResistance_kohm,BINP_outputs_50ms.BINP_BMS_FrP01.VINP_HVBattSOC_pct,BINP_outputs_50ms.BINP_BMS_FrP01.VINP_HVBattVoltage_V,BINP_outputs_50ms.BINP_BMS_FrP01.VINP_HVBattCurrent_A,BINP_outputs_50ms.BINP_BMS_FrP01.VINP_BMSHSC2FrP01Active_flg,BINP_outputs_50ms.BINP_BMS_HSC_FrP02.VINP_BMSMainRelayStat_enum,BINP_outputs_50ms.BINP_BMS_HSC_FrP02.VINP_HVBattCellTempMax_C,BINP_outputs_50ms.BINP_BMS_HSC_FrP02.VINP_HVBattChargerPlugged_flg,BINP_outputs_50ms.BINP_BMS_HSC_FrP02.VINP_HVBattChillerOffReq_flg,BINP_outputs_50ms.BINP_BMS_HSC_FrP02.VINP_HVBattCoolTemp_C,BINP_outputs_50ms.BINP_BMS_HSC_FrP02.VINP_HVBattCoolingPumpStatus_enum,BINP_outputs_50ms.BINP_BMS_HSC_FrP02.VINP_HVBattHVILClosed_flg,BINP_outputs_50ms.BINP_BMS_HSC_FrP02.VINP_HVBattBasicStatus_enum,BINP_outputs_20ms.BINP_BMS_HSC2_FrP09.VINP_HVBattPwrAvailCharge_kW,BINP_outputs_20ms.BINP_BMS_HSC2_FrP09.VINP_HVBattPwrAvailDischarge_kW,BINP_outputs_50ms.BINP_BMS_HSC_FrP02.VINP_BMSHSC2FrP02Active_flg,BINP_outputs_100ms.BINP_ISC_HSC2_FrP05.VINP_ISGInverterTemp_C,BINP_outputs_100ms.BINP_ISC_HSC2_FrP05.VINP_ISGMotorTemp_C,BINP_outputs_100ms.BINP_ISC_HSC2_FrP05.VINP_ISGRotorTemp_C,BINP_outputs_100ms.BINP_ISC_HSC2_FrP05.VINP_ISGPwrAct_kW,BINP_outputs_100ms.BINP_ISC_HSC2_FrP05.VINP_ISGOffsetAng_deg,BINP_outputs_100ms.BINP_ISC_HSC2_FrP05.VINP_ISGPumpStatus_enum,BINP_outputs_100ms.BINP_ISC_HSC2_FrP05.VINP_ISGFltLampOnReq_flg,BINP_outputs_100ms.BINP_ISC_HSC2_FrP05.VINP_ISGInhibitHV_flg,BINP_outputs_100ms.BINP_ISC_HSC2_FrP05.VINP_ISCHSC2FrP05Active_flg,BINP_outputs_100ms.BINP_TC_HSC2_FrP03.VINP_TMInverterTemp_C,BINP_outputs_100ms.BINP_TC_HSC2_FrP03.VINP_TMMotorTemp_C,BINP_outputs_100ms.BINP_TC_HSC2_FrP03.VINP_TMRotorTemp_C,BINP_outputs_100ms.BINP_TC_HSC2_FrP03.VINP_TMPwrAct_kW,BINP_outputs_100ms.BINP_TC_HSC2_FrP03.VINP_TMOffsetAng_deg,BINP_outputs_100ms.BINP_TC_HSC2_FrP03.VINP_TMFltLampOnReq_flg,BINP_outputs_100ms.BINP_TC_HSC2_FrP03.VINP_TMInhibitHV_flg,BINP_outputs_100ms.BINP_TC_HSC2_FrP03.VINP_TCHSC2FrP03Active_flg,BINP_outputs_100ms.BINP_ISC_HSC2_FrP01.VINP_DCDCHVCurr_A,BINP_outputs_100ms.BINP_ISC_HSC2_FrP01.VINP_DCDCHVVolt_V,BINP_outputs_100ms.BINP_ISC_HSC2_FrP01.VINP_DCDCLVCurr_A,BINP_outputs_100ms.BINP_ISC_HSC2_FrP01.VINP_DCDCLVVolt_V,BINP_outputs_100ms.BINP_ISC_HSC2_FrP01.VINP_DCDCOpMode_enum,BINP_outputs_100ms.BINP_ISC_HSC2_FrP01.VINP_HVAccessoryPower_kW,BINP_outputs_100ms.BINP_ISC_HSC2_FrP01.VINP_ISCHSC2FrP01Active_flg,BINP_outputs_100ms.BINP_ISC_HSC2_FrP02.VINP_DCDCFault_flg,BINP_outputs_100ms.BINP_ISC_HSC2_FrP02.VINP_DCDCTemp_C,BINP_outputs_100ms.BINP_ISC_HSC2_FrP02.VINP_DCDCLVLoad_pct,BINP_outputs_100ms.BINP_ISC_HSC2_FrP02.VINP_ISCHSC2FrP02Active_flg,BINP_outputs_100ms.BINP_PMU_HSC_FrP00.VINP_DCDCVoltSetpt_V,BINP_outputs_100ms.BINP_PMU_HSC_FrP00.VINP_PMUHSCFrP00Active_flg,BINP_outputs_100ms.BINP_SMU_HSC_FrP06.VINP_DriverDoorOpen_flg,BINP_outputs_100ms.BINP_SMU_HSC_FrP06.VINP_BonnetOpen_flg,BINP_outputs_100ms.BINP_SMU_HSC_FrP06.VINP_ATCEngOnReq_enum,BINP_outputs_100ms.BINP_SMU_HSC_FrP06.VINP_ACCompressorPower_kW,BINP_outputs_100ms.BINP_SMU_HSC_FrP06.VINP_SMUHSCFrP06Active_flg,BINP_outputs_100ms.BINP_SMU_HSC_FrP07.VINP_SteerLockEngaged_flg,BINP_outputs_100ms.BINP_SMU_HSC_FrP07.VINP_SMUHSCFrP07Active_flg,BINP_outputs_100ms.BINP_SMU_HSC_FrP00.VINP_ATCACOn_flg,BINP_outputs_100ms.BINP_SMU_HSC_FrP00.VINP_FuelLevel_L,BINP_outputs_100ms.BINP_SMU_HSC_FrP00.VINP_FuelLevelValid_flg,BINP_outputs_100ms.BINP_SMU_HSC_FrP00.VINP_SMUHSCFrP00Active_flg,BINP_outputs_100ms.BINP_HW_HCU_100ms.VINP_EDUCoolantTemp_C,BINP_outputs_100ms.BINP_HW_HCU_100ms.VINP_EDUCoolantTempValid_flg,BINP_outputs_100ms.BINP_HW_HCU_100ms.VINP_EDUOilTemp_C,BINP_outputs_100ms.BINP_HW_HCU_100ms.VINP_EDUOilTempValid_flg,BINP_outputs_100ms.BINP_HW_HCU_100ms.VINP_VehMode_enum,BINP_outputs_10ms.BINP_EMS_HSC_FrP00.VINP_BrkLightSWPUnlockActive_flg,BINP_outputs_10ms.BINP_EMS_HSC_FrP00.VINP_BrkLightSWPUnlockActiveValid_flg,BINP_outputs_5ms.VINP_EDUOutputShaftSpdRawValid_flg,BINP_outputs_10ms.BINP_ABS_DSC_HSC_FrP00.VINP_VehSpdRawValid_flg,BINP_outputs_100ms.BINP_ISC_HSC2_FrP02.VINP_ISGDerating_flg,BINP_outputs_100ms.BINP_ISC_HSC2_FrP02.VINP_ISGOverTemp_flg,BINP_outputs_10ms.BINP_TC_HSC2_FrP01.VINP_TMDerating_flg,BINP_outputs_10ms.BINP_TC_HSC2_FrP01.VINP_TMOverTemp_flg,BINP_outputs_10ms.BINP_SCU_HSC_FrP00.VINP_ShifterPosProtFault_flg,BINP_outputs_20ms.BINP_BMS_HSC2_FrP09.VINP_BMSPeakChrgPwr_kW,BINP_outputs_20ms.BINP_BMS_HSC2_FrP09.VINP_BMSPeakChrgPwrVld_flg,BINP_outputs_20ms.BINP_BMS_HSC2_FrP09.VINP_BMSPeakDchaPwr_kW,BINP_outputs_20ms.BINP_BMS_HSC2_FrP09.VINP_BMSPeakDchaPwrVld_flg,BINP_outputs_20ms.BINP_BMS_HSC2_FrP09.VINP_BMSChrgBuffer_pct,BINP_outputs_20ms.BINP_BMS_HSC2_FrP09.VINP_BMSDchaBuffer_pct,BINP_outputs_50ms.BINP_BMS_HSC_FrP05.VINP_BMSCellTempMin_C,BINP_outputs_50ms.BINP_BMS_HSC_FrP05.VINP_BMSPackSOCDisp_pct,BINP_outputs_50ms.BINP_BMS_HSC_FrP02.VINP_BMSColdCrkCtrl_enum,BINP_outputs_20ms.BINP_HW_HCU_20ms.VINP_EDUOilPressure_bar,BINP_outputs_20ms.BINP_HW_HCU_20ms.VINP_EDUOilPressureValid_flg  OutputAsBus=on
  Bus Selector9 : BusSelector  OutputSignals=VDSM_SngAccPedInvldFlt_flg
  BINP_outputs : Outport  UseBusObject=on  OutDataType=fixdt(1, 16)  OutScaling=2^0
      settings: BusObject=BINP_outputs
  wires:
  Bus Selector9/1 -> BINP_ouputs_10ms/5(VDSM_SngAccPedInvldFlt_flg)  "<VDSM_SngAccPedInvldFlt_flg>"
  BDSM_outputs/1 -> Bus Selector9/1
  Bus Selector/3 -> [trig_sig_chk_100ms]  "<trig_sig_chk_100ms>"
  Bus Selector/2 -> [trig_sig_chk_10ms]  "<trig_sig_chk_10ms>"
  Bus Selector/1 -> [trig_sig_chk_5ms]  "<trig_sig_chk_5ms>"
  trig_sig_chk/1 -> Bus Selector/1
  [VINP_VehSpdValid_flg] -> BINP_ouputs_10ms/3(VINP_VehSpdValid_flg)
  [VINP_VehSpd_kph] -> BINP_ouputs_10ms/2(VINP_VehSpd_kph)
  [trig_sig_chk_10ms] -> BINP_ouputs_10ms/1(trig_sig_chk_10ms)
  BINP_ouputs_5ms/3(VINP_VehSpdValid_flg) -> [VINP_VehSpdValid_flg]
  BINP_ouputs_100ms/1(BINP_outputs_100ms) -> Bus Creator/5
  [VINP_VehSpd_kph] -> BINP_ouputs_100ms/2(VINP_VehSpd_kph)
  Bus Selector5/1 -> BINP_ouputs_100ms/3(BINP_rawoutputs_100ms)  "BINP_rawoutputs_100ms"
  [trig_sig_chk_100ms] -> BINP_ouputs_100ms/1(trig_sig_chk)
  [trig_sig_chk_5ms] -> BINP_ouputs_5ms/1(trig_sig_chk)
  BINP_ouputs_5ms/1(BINP_outputs_5ms) -> Bus Creator/1
  BINP_ouputs_5ms/2(VINP_VehSpd_kph) -> [VINP_VehSpd_kph]
  BINP_rawoutputs/1 -> Bus Selector2/1, Bus Selector5/1, Bus Selector4/1, Bus Selector3/1, Bus Selector1/1, Bus Selector6/1
  Bus Creator/1 -> Bus Selector7/1
  Bus Selector6/1 -> BINP_ouputs_5ms/2(BINP_rawoutputs_5ms)  "<BINP_rawoutputs_5ms>"
  Bus Selector4/1 -> Bus Creator/4  "BINP_outputs_50ms"
  BINP_ouputs_10ms/1(BINP_outputs_10ms) -> Bus Creator/2
  Bus Selector1/1 -> BINP_ouputs_5ms/3(BINP_rawoutputs_10ms)  "<BINP_rawoutputs_10ms>"
  Bus Selector2/1 -> BINP_ouputs_10ms/4(BINP_rawoutputs_10ms)
  Bus Selector7/1 -> BINP_outputs/1  "BINP_outputs"
  Bus Selector3/1 -> Bus Creator/3  "BINP_outputs_20ms"

== system inp/INP/Version_Control ==
  note: 2013-05-17 11:23:56: 11.0.27 by tunfl
  note: 2013-04-10 13:17:51: 11.0.24 by wuqnj
  note: 2013-03-19 10:42:23: 11.0.21 by wuqnj
  note: 2013-03-18 18:27:34: 11.0.20 by wuqnj
  note: Model change history list, Detailed model change log can be found in "Model History":
  note: 2012-08-28 16:30:24: 11.0.9 by tunfl
  note: 2012-09-03 11:55:18: 11.0.10 by tunfl
  note: 2012-10-10 16:30:31: 11.0.11 by tunfl
  note: 2012-10-11 11:20:51: 11.0.12 by tunfl
  note: 2012-10-11 11:22:44: 11.0.13 by tunfl
  note: 2012-10-16 14:48:04: 11.0.14 by tunfl
  note: 2012-10-19 16:16:11: 11.0.15 by tunfl
  note: 2012-11-23 11:36:28: 11.0.16 by tunfl
  note: 2012-12-04 09:11:36: 11.0.17 by tunfl
  note: 2013-03-15 10:45:21: 11.0.18 by wuqnj
  note: 2013-03-19 10:45:50: 11.0.22 by wuqnj
  note: 2013-04-10 13:18:30: 11.0.25 by wuqnj
  note: 2013-04-22 16:40:45: 11.0.26 by tunfl
  note: 2013-07-25 13:52:57: 11.0.28 by tunfl
  note: 2013-08-02 09:13:15: 11.0.29 by tunfl
  note: 2013-08-05 11:11:04: 11.0.30 by tunfl
  Submit : Subsystem  mask{temp=0}
      settings: OpenFcn=seat_version_control_block_callbacks(get_param(gcb,'Parent'),'submit')
      mask Display: disp(sprintf('Double click to save and \nsubmit version update'))
